simulink model "mdl_4reac_2pump_arduino"  (R2020b)
settings: Solver=FixedStepAuto  StartTime=0.0  StopTime=1000  FixedStep=h  MaxStep=1  RelTol=1e-3  AbsTol=1e-6
undefined symbols (not defined in the file): p_4reac_2pump
settings Model: SILPILModeSetting=veronly  PacingRate=0.100000  ExtModeTrigDuration=2  Creator=nobel  LastModifiedBy=natha
settings OptimizationCC: EnhancedBackFolding=on  PassReuseOutputArgsAs=Individual arguments  ZeroExternalMemoryAtStartup=off  ZeroInternalMemoryAtStartup=off  MaxStackSize=64  OptimizeBlockOrder=speed  DifferentSizesBufferReuse=on  OptimizationCustomize=off  EfficientTunableParamExpr=on
settings DebuggingCC: ParameterTunabilityLossMsg=error
settings HardwareCC: ProdBitPerInt=16  ProdBitPerPointer=16  ProdBitPerSizeT=16  ProdBitPerPtrDiffT=16  ProdLargestAtomicFloat=None  ProdWordSize=8  ProdHWDeviceType=Atmel->AVR  UseEmbeddedCoderFeatures=off  UseSimulinkCoderFeatures=off
settings SFSimCC: MATLABDynamicMemAlloc=off
settings RTWCC: Description=Embedded Coder  SystemTargetFile=ert.tlc  HardwareBoard=Arduino Mega 2560  TemplateMakefile=ert_default_tmf  Toolchain=Arduino AVR
settings CodeAppCC: ForceParamTrailComments=on  IgnoreCustomStorageClasses=off  OperatorAnnotations=on  SimulinkDataObjDesc=on  SFDataObjDesc=on  InsertBlockDesc=on
settings ERTTargetCC: SupportContinuousTime=on  SupportNonInlinedSFcns=on  SupportVariableSizeSignals=on  ExtModeStaticAllocSize=2048

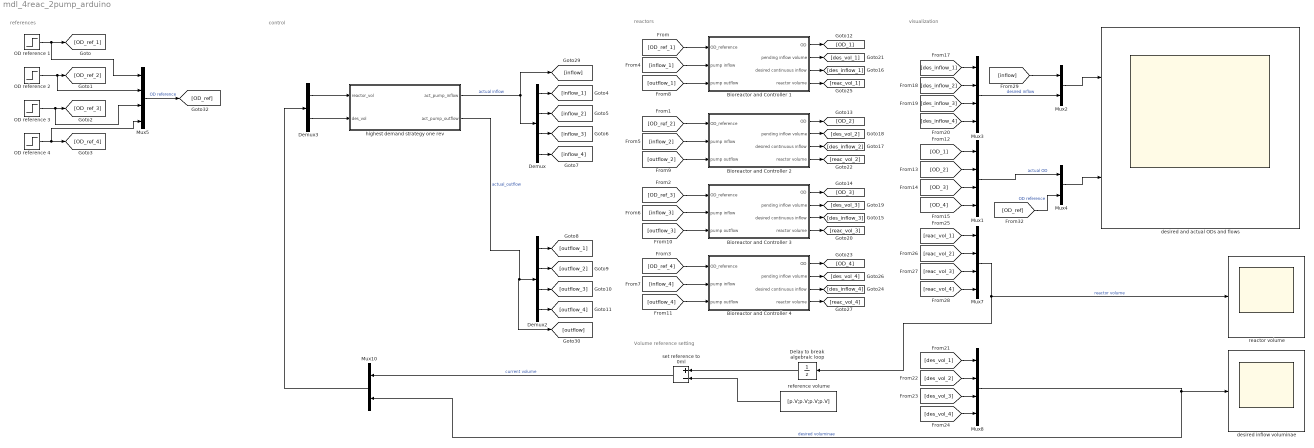
== system mdl_4reac_2pump_arduino ==
  note: control
  note: Volume reference setting
  note: visualization
  note: reactors
  note: references
  Bioreactor and Controller 1 : Subsystem  mask{p=p_4reac_2pump}
      mask prompts: p "Reactor Parameter Struct"
  Bioreactor and Controller 2 : Subsystem  mask{p=p_4reac_2pump}
      mask prompts: p "Reactor Parameter Struct"
  Bioreactor and Controller 3 : Subsystem  mask{p=p_4reac_2pump}
      mask prompts: p "Reactor Parameter Struct"
  Bioreactor and Controller 4 : Subsystem  mask{p=p_4reac_2pump}
      mask prompts: p "Reactor Parameter Struct"
  Delay to break algebraic loop : UnitDelay  InitialCondition=[15; 15; 15; 15]  SampleTime=-1  HasFrameUpgradeWarning=on
  Demux : Demux
  Demux2 : Demux
  Demux3 : Demux  Outputs=2
  Mux{1,3,5,7..8} (5 alike) : Mux
  Mux10 : Mux  Inputs=2
  Mux2 : Mux  Inputs=2
  Mux4 : Mux  Inputs=2
  OD reference 1 : Step  Time=p.r1.step_time  Before=p.r1.init_val  After=p.r1.final_val  SampleTime=0  mask{p=p_4reac_2pump}
      mask prompts: p "Reactor Parameter Struct"
  OD reference 2 : Step  Time=p.r2.step_time  Before=p.r2.init_val  After=p.r2.final_val  SampleTime=0  mask{p=p_4reac_2pump}
      mask prompts: p "Reactor Parameter Struct"
  OD reference 3 : Step  Time=p.r3.step_time  Before=p.r3.init_val  After=p.r3.final_val  SampleTime=0  mask{p=p_4reac_2pump}
      mask prompts: p "Reactor Parameter Struct"
  OD reference 4 : Step  Time=p.r4.step_time  Before=p.r4.init_val  After=p.r4.final_val  SampleTime=0  mask{p=p_4reac_2pump}
      mask prompts: p "Reactor Parameter Struct"
  desired and actual ODs and flows : Scope  NumInputPorts=2
  desired inflow voluminae : Scope
  highest demand strategy one rev : Stateflow chart  TreatAsAtomicUnit=on  mask{p=p_4reac_2pump}
      mask prompts: p "Reactor Parameter Struct"
  reactor volume : Scope
  reference volume : Constant  Value=[p.V;p.V;p.V;p.V]  mask{p=p_4reac_2pump}
      mask prompts: p "Reactor Parameter Struct"
  set reference to 0ml : Sum  Inputs=+-
  wires:
  Bioreactor and Controller 1/2(pending inflow volume) -> [des_vol_1]
  Mux8/1 -> Mux10/2, desired inflow voluminae/1  "desired voluminae"
  Mux1/1 -> Mux4/1  "actual OD"
  Mux2/1 -> desired and actual ODs and flows/1
  Mux3/1 -> Mux2/2  "desired inflow"
  Mux4/1 -> desired and actual ODs and flows/2
  Mux5/1 -> [OD_ref]  "OD reference"
  highest demand strategy one rev/1(act_pump_inflow) -> Demux/1, [inflow]  "actual inflow"
  Mux7/1 -> Delay to break algebraic loop/1, reactor volume/1  "reactor volume"
  reference volume/1 -> set reference to 0ml/2
  OD reference 1/1 -> Mux5/1, [OD_ref_1]
  OD reference 2/1 -> Mux5/2, [OD_ref_2]
  OD reference 3/1 -> Mux5/3, [OD_ref_3]
  OD reference 4/1 -> Mux5/4, [OD_ref_4]
  [OD_ref_1] -> Bioreactor and Controller 1/1(OD_reference)
  [OD_ref_2] -> Bioreactor and Controller 2/1(OD_reference)
  [OD_ref_3] -> Bioreactor and Controller 3/1(OD_reference)
  [OD_ref_4] -> Bioreactor and Controller 4/1(OD_reference)
  Demux/1 -> [inflow_1]
  Demux/2 -> [inflow_2]
  Demux/3 -> [inflow_3]
  Demux/4 -> [inflow_4]
  [inflow_1] -> Bioreactor and Controller 1/2(pump inflow)
  [inflow_2] -> Bioreactor and Controller 2/2(pump inflow)
  [inflow_3] -> Bioreactor and Controller 3/2(pump inflow)
  [inflow_4] -> Bioreactor and Controller 4/2(pump inflow)
  Demux2/4 -> [outflow_4]
  Demux2/3 -> [outflow_3]
  Demux2/2 -> [outflow_2]
  Demux2/1 -> [outflow_1]
  [outflow_1] -> Bioreactor and Controller 1/3(pump outflow)
  [outflow_2] -> Bioreactor and Controller 2/3(pump outflow)
  [outflow_3] -> Bioreactor and Controller 3/3(pump outflow)
  [outflow_4] -> Bioreactor and Controller 4/3(pump outflow)
  Bioreactor and Controller 1/1(OD) -> [OD_1]
  [OD_1] -> Mux1/1
  [OD_2] -> Mux1/2
  [OD_3] -> Mux1/3
  [OD_4] -> Mux1/4
  [des_inflow_1] -> Mux3/1
  [des_inflow_2] -> Mux3/2
  [des_inflow_3] -> Mux3/3
  [des_inflow_4] -> Mux3/4
  [des_vol_4] -> Mux8/4
  [des_vol_3] -> Mux8/3
  [des_vol_2] -> Mux8/2
  [des_vol_1] -> Mux8/1
  Bioreactor and Controller 1/4(reactor volume) -> [reac_vol_1]
  [reac_vol_1] -> Mux7/1
  [reac_vol_2] -> Mux7/2
  [reac_vol_3] -> Mux7/3
  [reac_vol_4] -> Mux7/4
  highest demand strategy one rev/2(act_pump_outflow) -> [outflow], Demux2/1  "actual_outflow"
  [inflow] -> Mux2/1
  [OD_ref] -> Mux4/2  "OD reference"
  set reference to 0ml/1 -> Mux10/1  "current volume"
  Delay to break algebraic loop/1 -> set reference to 0ml/1
  Bioreactor and Controller 1/3(desired continuous inflow) -> [des_inflow_1]
  Bioreactor and Controller 2/3(desired continuous inflow) -> [des_inflow_2]
  Bioreactor and Controller 2/4(reactor volume) -> [reac_vol_2]
  Bioreactor and Controller 2/1(OD) -> [OD_2]
  Bioreactor and Controller 2/2(pending inflow volume) -> [des_vol_2]
  Bioreactor and Controller 3/2(pending inflow volume) -> [des_vol_3]
  Bioreactor and Controller 3/1(OD) -> [OD_3]
  Bioreactor and Controller 3/4(reactor volume) -> [reac_vol_3]
  Bioreactor and Controller 3/3(desired continuous inflow) -> [des_inflow_3]
  Bioreactor and Controller 4/3(desired continuous inflow) -> [des_inflow_4]
  Bioreactor and Controller 4/4(reactor volume) -> [reac_vol_4]
  Bioreactor and Controller 4/1(OD) -> [OD_4]
  Bioreactor and Controller 4/2(pending inflow volume) -> [des_vol_4]
  Demux3/1 -> highest demand strategy one rev/1(reactor_vol)
  Demux3/2 -> highest demand strategy one rev/2(des_vol)
  Mux10/1 -> Demux3/1

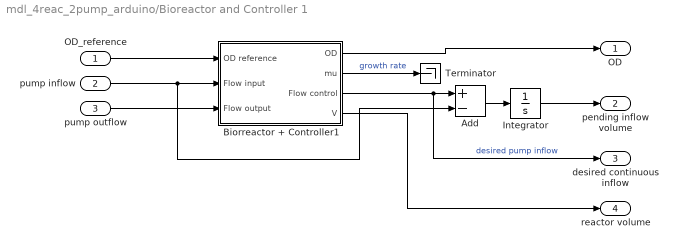
== system mdl_4reac_2pump_arduino/Bioreactor and Controller 1 ==
  OD_reference : Inport
  pump inflow : Inport  Port=2
  pump outflow : Inport  Port=3
  Add : Sum  Inputs=+-
  Biorreactor + Controller1 : Subsystem
  Integrator : Integrator
  Terminator : Terminator
  OD : Outport
  pending inflow volume : Outport  Port=2
  desired continuous inflow : Outport  Port=3
  reactor volume : Outport  Port=4
  wires:
  OD_reference/1 -> Biorreactor + Controller1/1(OD reference)
  Biorreactor + Controller1/2(mu) -> Terminator/1  "growth rate"
  Biorreactor + Controller1/1(OD) -> OD/1
  Biorreactor + Controller1/3(Flow control) -> desired continuous inflow/1, Add/1  "desired pump inflow"
  pump inflow/1 -> Add/2, Biorreactor + Controller1/2(Flow input)
  Biorreactor + Controller1/4(V) -> reactor volume/1
  pump outflow/1 -> Biorreactor + Controller1/3(Flow output)
  Add/1 -> Integrator/1
  Integrator/1 -> pending inflow volume/1

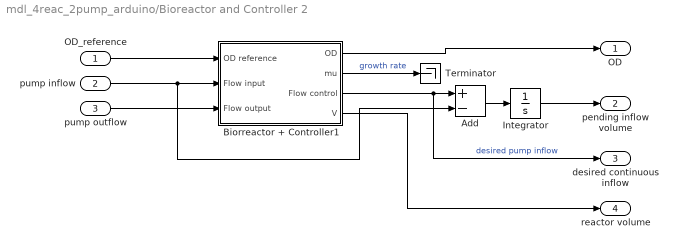
== system mdl_4reac_2pump_arduino/Bioreactor and Controller 2 ==
  OD_reference : Inport
  pump inflow : Inport  Port=2
  pump outflow : Inport  Port=3
  Add : Sum  Inputs=+-
  Biorreactor + Controller1 : Subsystem
  Integrator : Integrator
  Terminator : Terminator
  OD : Outport
  pending inflow volume : Outport  Port=2
  desired continuous inflow : Outport  Port=3
  reactor volume : Outport  Port=4
  wires:
  Integrator/1 -> pending inflow volume/1
  Add/1 -> Integrator/1
  pump outflow/1 -> Biorreactor + Controller1/3(Flow output)
  Biorreactor + Controller1/4(V) -> reactor volume/1
  pump inflow/1 -> Biorreactor + Controller1/2(Flow input), Add/2
  Biorreactor + Controller1/3(Flow control) -> Add/1, desired continuous inflow/1  "desired pump inflow"
  Biorreactor + Controller1/1(OD) -> OD/1
  Biorreactor + Controller1/2(mu) -> Terminator/1  "growth rate"
  OD_reference/1 -> Biorreactor + Controller1/1(OD reference)

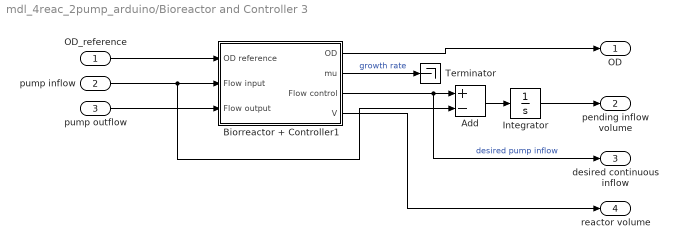
== system mdl_4reac_2pump_arduino/Bioreactor and Controller 3 ==
  OD_reference : Inport
  pump inflow : Inport  Port=2
  pump outflow : Inport  Port=3
  Add : Sum  Inputs=+-
  Biorreactor + Controller1 : Subsystem
  Integrator : Integrator
  Terminator : Terminator
  OD : Outport
  pending inflow volume : Outport  Port=2
  desired continuous inflow : Outport  Port=3
  reactor volume : Outport  Port=4
  wires:
  OD_reference/1 -> Biorreactor + Controller1/1(OD reference)
  Biorreactor + Controller1/2(mu) -> Terminator/1  "growth rate"
  Biorreactor + Controller1/1(OD) -> OD/1
  Biorreactor + Controller1/3(Flow control) -> desired continuous inflow/1, Add/1  "desired pump inflow"
  pump inflow/1 -> Add/2, Biorreactor + Controller1/2(Flow input)
  Biorreactor + Controller1/4(V) -> reactor volume/1
  pump outflow/1 -> Biorreactor + Controller1/3(Flow output)
  Add/1 -> Integrator/1
  Integrator/1 -> pending inflow volume/1

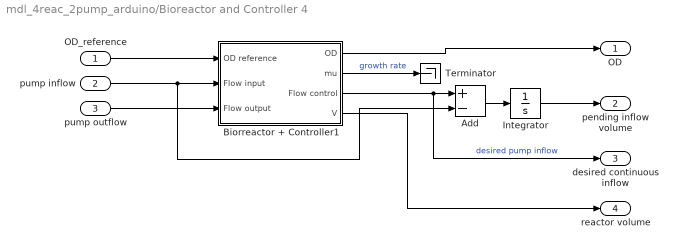
== system mdl_4reac_2pump_arduino/Bioreactor and Controller 4 ==
  OD_reference : Inport
  pump inflow : Inport  Port=2
  pump outflow : Inport  Port=3
  Add : Sum  Inputs=+-
  Biorreactor + Controller1 : Subsystem
  Integrator : Integrator
  Terminator : Terminator
  OD : Outport
  pending inflow volume : Outport  Port=2
  desired continuous inflow : Outport  Port=3
  reactor volume : Outport  Port=4
  wires:
  Integrator/1 -> pending inflow volume/1
  Add/1 -> Integrator/1
  pump outflow/1 -> Biorreactor + Controller1/3(Flow output)
  Biorreactor + Controller1/4(V) -> reactor volume/1
  pump inflow/1 -> Biorreactor + Controller1/2(Flow input), Add/2
  Biorreactor + Controller1/3(Flow control) -> Add/1, desired continuous inflow/1  "desired pump inflow"
  Biorreactor + Controller1/1(OD) -> OD/1
  Biorreactor + Controller1/2(mu) -> Terminator/1  "growth rate"
  OD_reference/1 -> Biorreactor + Controller1/1(OD reference)

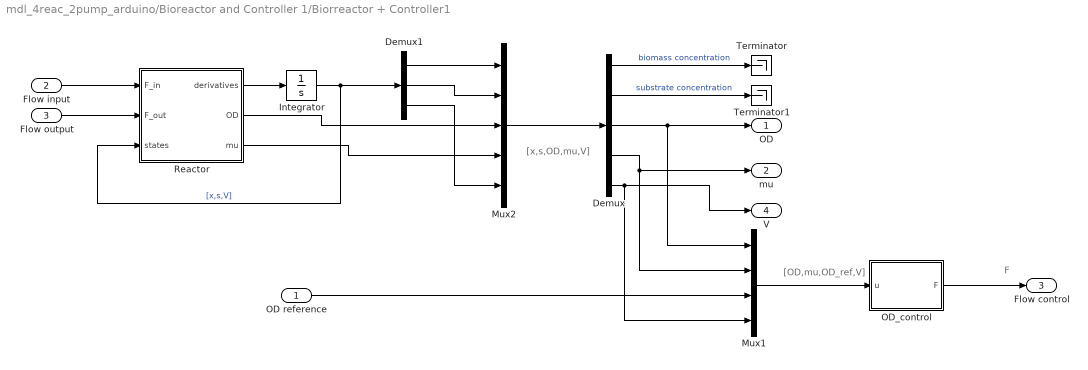
== system mdl_4reac_2pump_arduino/Bioreactor and Controller 1/Biorreactor + Controller1 ==
  note: [OD,mu,OD_ref,V]
  note: F
  note: [x,s,OD,mu,V]
  OD reference : Inport
  Flow input : Inport  Port=2
  Flow output : Inport  Port=3
  Demux : Demux  Outputs=5
  Demux1 : Demux  Outputs=3
  Integrator : Integrator  InitialCondition=[0.1 16 15]
  Mux1 : Mux
  Mux2 : Mux  Inputs=5
  OD_control : MATLAB Function  TreatAsAtomicUnit=on
  Reactor : MATLAB Function  TreatAsAtomicUnit=on
  Terminator : Terminator
  Terminator1 : Terminator
  OD : Outport
  mu : Outport  Port=2
  Flow control : Outport  Port=3
  V : Outport  Port=4
  wires:
  Demux/4 -> Mux1/2, mu/1
  Demux/3 -> Mux1/1, OD/1
  OD reference/1 -> Mux1/3
  Mux2/1 -> Demux/1
  Demux/2 -> Terminator1/1  "substrate concentration"
  Mux1/1 -> OD_control/1(u)
  OD_control/1(F) -> Flow control/1
  Demux/1 -> Terminator/1  "biomass concentration"
  Demux/5 -> Mux1/4, V/1
  Flow output/1 -> Reactor/2(F_out)
  Reactor/1(derivatives) -> Integrator/1
  Integrator/1 -> Demux1/1, Reactor/3(states)  "[x,s,V]"
  Demux1/1 -> Mux2/1
  Demux1/2 -> Mux2/2
  Demux1/3 -> Mux2/5
  Reactor/2(OD) -> Mux2/3
  Reactor/3(mu) -> Mux2/4
  Flow input/1 -> Reactor/1(F_in)

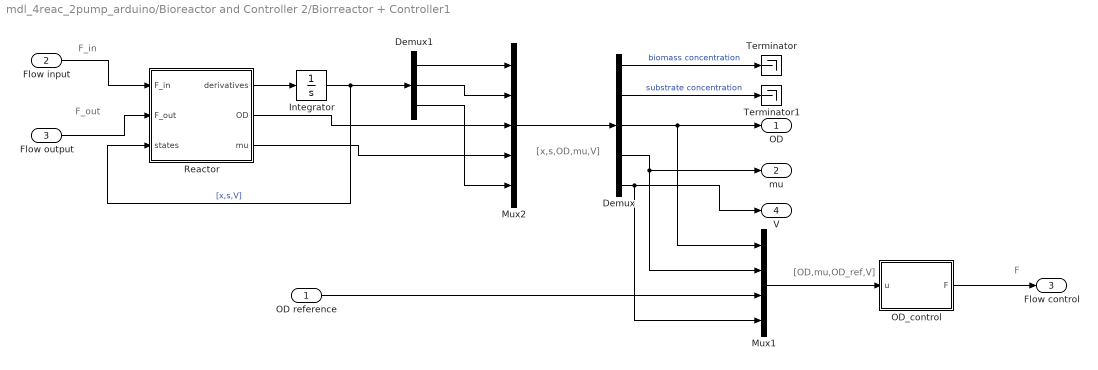
== system mdl_4reac_2pump_arduino/Bioreactor and Controller 2/Biorreactor + Controller1 ==
  note: F_in
  note: [x,s,OD,mu,V]
  note: F
  note: [OD,mu,OD_ref,V]
  note: F_out
  OD reference : Inport
  Flow input : Inport  Port=2
  Flow output : Inport  Port=3
  Demux : Demux  Outputs=5
  Demux1 : Demux  Outputs=3
  Integrator : Integrator  InitialCondition=[0.1 16 15]
  Mux1 : Mux
  Mux2 : Mux  Inputs=5
  OD_control : MATLAB Function  TreatAsAtomicUnit=on
  Reactor : MATLAB Function  TreatAsAtomicUnit=on
  Terminator : Terminator
  Terminator1 : Terminator
  OD : Outport
  mu : Outport  Port=2
  Flow control : Outport  Port=3
  V : Outport  Port=4
  wires:
  Flow input/1 -> Reactor/1(F_in)
  Reactor/3(mu) -> Mux2/4
  Reactor/2(OD) -> Mux2/3
  Demux1/3 -> Mux2/5
  Demux1/2 -> Mux2/2
  Demux1/1 -> Mux2/1
  Integrator/1 -> Reactor/3(states), Demux1/1  "[x,s,V]"
  Reactor/1(derivatives) -> Integrator/1
  Flow output/1 -> Reactor/2(F_out)
  Demux/5 -> V/1, Mux1/4
  Demux/1 -> Terminator/1  "biomass concentration"
  OD_control/1(F) -> Flow control/1
  Mux1/1 -> OD_control/1(u)
  Demux/2 -> Terminator1/1  "substrate concentration"
  Mux2/1 -> Demux/1
  OD reference/1 -> Mux1/3
  Demux/3 -> OD/1, Mux1/1
  Demux/4 -> mu/1, Mux1/2

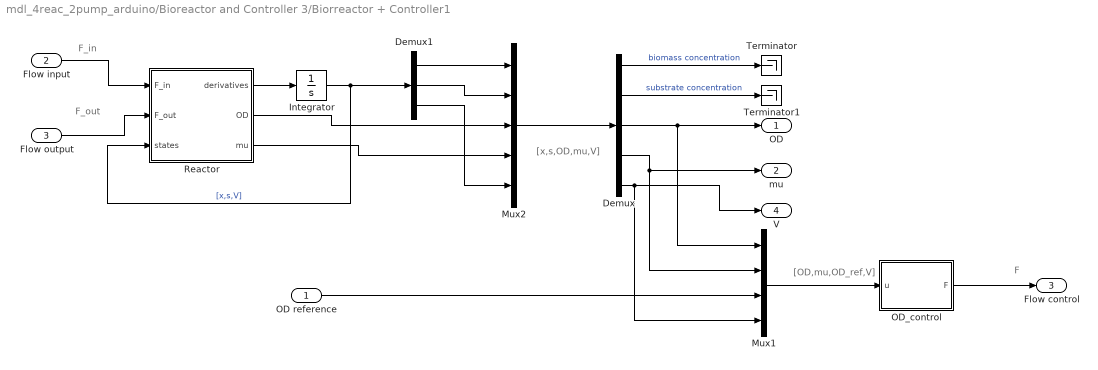
== system mdl_4reac_2pump_arduino/Bioreactor and Controller 3/Biorreactor + Controller1 ==
  note: F_out
  note: [OD,mu,OD_ref,V]
  note: F
  note: [x,s,OD,mu,V]
  note: F_in
  OD reference : Inport
  Flow input : Inport  Port=2
  Flow output : Inport  Port=3
  Demux : Demux  Outputs=5
  Demux1 : Demux  Outputs=3
  Integrator : Integrator  InitialCondition=[0.1 16 15]
  Mux1 : Mux
  Mux2 : Mux  Inputs=5
  OD_control : MATLAB Function  TreatAsAtomicUnit=on
  Reactor : MATLAB Function  TreatAsAtomicUnit=on
  Terminator : Terminator
  Terminator1 : Terminator
  OD : Outport
  mu : Outport  Port=2
  Flow control : Outport  Port=3
  V : Outport  Port=4
  wires:
  Demux/4 -> Mux1/2, mu/1
  Demux/3 -> Mux1/1, OD/1
  OD reference/1 -> Mux1/3
  Mux2/1 -> Demux/1
  Demux/2 -> Terminator1/1  "substrate concentration"
  Mux1/1 -> OD_control/1(u)
  OD_control/1(F) -> Flow control/1
  Demux/1 -> Terminator/1  "biomass concentration"
  Demux/5 -> Mux1/4, V/1
  Flow output/1 -> Reactor/2(F_out)
  Reactor/1(derivatives) -> Integrator/1
  Integrator/1 -> Demux1/1, Reactor/3(states)  "[x,s,V]"
  Demux1/1 -> Mux2/1
  Demux1/2 -> Mux2/2
  Demux1/3 -> Mux2/5
  Reactor/2(OD) -> Mux2/3
  Reactor/3(mu) -> Mux2/4
  Flow input/1 -> Reactor/1(F_in)

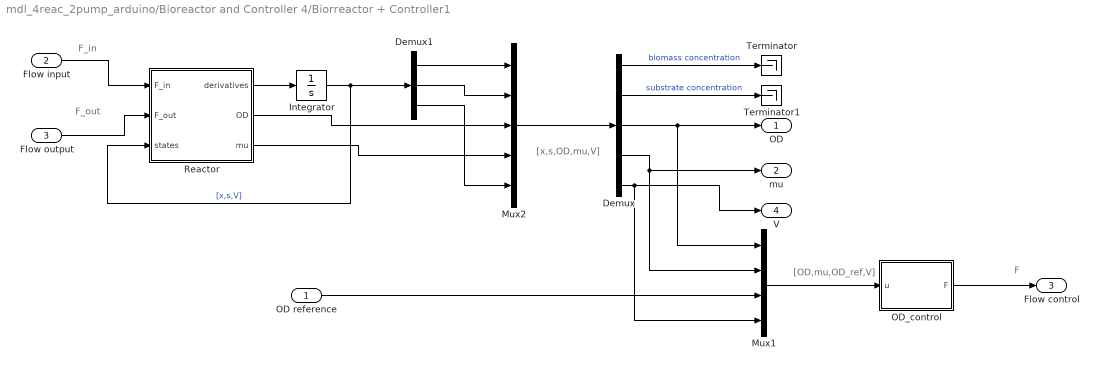
== system mdl_4reac_2pump_arduino/Bioreactor and Controller 4/Biorreactor + Controller1 ==
  note: F_in
  note: [x,s,OD,mu,V]
  note: F
  note: [OD,mu,OD_ref,V]
  note: F_out
  OD reference : Inport
  Flow input : Inport  Port=2
  Flow output : Inport  Port=3
  Demux : Demux  Outputs=5
  Demux1 : Demux  Outputs=3
  Integrator : Integrator  InitialCondition=[0.1 16 15]
  Mux1 : Mux
  Mux2 : Mux  Inputs=5
  OD_control : MATLAB Function  TreatAsAtomicUnit=on
  Reactor : MATLAB Function  TreatAsAtomicUnit=on
  Terminator : Terminator
  Terminator1 : Terminator
  OD : Outport
  mu : Outport  Port=2
  Flow control : Outport  Port=3
  V : Outport  Port=4
  wires:
  Flow input/1 -> Reactor/1(F_in)
  Reactor/3(mu) -> Mux2/4
  Reactor/2(OD) -> Mux2/3
  Demux1/3 -> Mux2/5
  Demux1/2 -> Mux2/2
  Demux1/1 -> Mux2/1
  Integrator/1 -> Reactor/3(states), Demux1/1  "[x,s,V]"
  Reactor/1(derivatives) -> Integrator/1
  Flow output/1 -> Reactor/2(F_out)
  Demux/5 -> V/1, Mux1/4
  Demux/1 -> Terminator/1  "biomass concentration"
  OD_control/1(F) -> Flow control/1
  Mux1/1 -> OD_control/1(u)
  Demux/2 -> Terminator1/1  "substrate concentration"
  Mux2/1 -> Demux/1
  OD reference/1 -> Mux1/3
  Demux/3 -> OD/1, Mux1/1
  Demux/4 -> mu/1, Mux1/2

== stateflow chart mdl_4reac_2pump_arduino/highest demand strategy one rev ==
  state procedures [parallel]
    settings: executionOrder=1
    state normal
    state sampling
      entry: sampling_req=true;
    (default) -> normal
    normal -> sampling : after(15, sec)
    sampling -> normal : sampling_done
  state feeding [parallel]
    settings: executionOrder=2
    state inflow
      state inflow_act
        entry: act_pump_inflow(reac_ind_inflow)=...
        p.max_pump_flow;
      state inflow_inact
        entry: act_pump_inflow=zeros(4,1);
        [vol_pump_in, reac_ind_inflow] = max(des_vol);
        during: [vol_pump_in, reac_ind_inflow] = max(des_vol);
      inflow_act -> inflow_inact : after(p.pump_res/p.max_pump_flow,sec)
      inflow_inact -> inflow_act : [vol_pump_in>=p.pump_res]
    (default) -> inflow_inact
  state wasting_sampling [parallel]
    settings: executionOrder=3
    state outflow_waste
      state outflow_act
        entry: act_pump_outflow(reac_ind_outflow)=...
        p.max_pump_flow;
      state outflow_inact
        entry: act_pump_outflow=zeros(4,1);
        [vol_pump_out, reac_ind_outflow] = max(reactor_vol);
        during: [vol_pump_out, reac_ind_outflow] = ...
        max(reactor_vol);
      wasting_sampling.outflow_waste.outflow_act -> wasting_sampling.outflow_waste.outflow_inact [order 1] : after(vol_pump_out/p.max_pump_flow,sec)
      wasting_sampling.outflow_waste.outflow_act -> wasting_sampling.outflow_waste.outflow_inact [order 2] : [vol_pump_out<=0]
      wasting_sampling.outflow_waste.outflow_inact -> wasting_sampling.outflow_waste.outflow_act [order 2] : [vol_pump_out>=p.pump_res]
    state cleaning_procedure
    state outflow_sampling
      state outflow_act
        entry: vol_pump_out=p.pump_res;
        act_pump_outflow(reac_ind_outflow)=p.max_pump_flow;
      state outflow_inact
        entry: act_pump_outflow=zeros(4,1);
      wasting_sampling.outflow_sampling.outflow_act -> wasting_sampling.outflow_sampling.outflow_inact : after(vol_pump_out/p.max_pump_flow,sec)
      wasting_sampling.outflow_sampling.outflow_inact -> wasting_sampling.outflow_sampling.outflow_act [order 2] : {reac_ind_outflow=reac_ind_outflow+1;}
    (default) -> wasting_sampling.outflow_waste.outflow_inact
    wasting_sampling.outflow_waste.outflow_inact -> cleaning_procedure [order 1] : [in(procedures.sampling)]
    wasting_sampling.outflow_sampling.outflow_inact -> wasting_sampling.outflow_waste.outflow_inact [order 1] : [reac_ind_outflow==4]{send(sampling_done,procedures)}
    cleaning_procedure -> (junction 263) : after(p.clean_time,sec)
    (junction 263) -> wasting_sampling.outflow_sampling.outflow_act : {reac_ind_outflow=1;}
  data: act_pump_inflow output =[0;0;0;0]; reactor_vol input; des_vol input size=4; vol_pump_in local; act_pump_outflow output =[0;0;0;0]; vol_pump_out local; reac_ind_inflow local =1; sampling_req local; p parameter; reac_ind_outflow local =1
  events: sampling_done local FUNCTION_CALL_EVENT

== matlab function mdl_4reac_2pump_arduino/Bioreactor and Controller 1/Biorreactor + Controller1/Reactor ==
  data: F_in input; derivatives output; F_out input; states input; p parameter; OD output; mu output
function [derivatives, OD, mu] = fcn(F_in,F_out,states, p)

x=states(1);
s=states(2);
V=states(3);

D = F_in/V;
mu = p.mu_max*s/(p.K_s+s);

%dx    (Concentration of biomass in the biorreactor)
dx= mu*x - D*x;

%ds    (Concentration of substrate in the biorreactor)
ds= -p.y*mu*x + D*(p.s_f - s);

%dV    (Volume of liquid inside the biorreactor)
dV= F_in - F_out;

OD=x/p.m_p/p.nOD;


derivatives = [dx ds dV];

== matlab function mdl_4reac_2pump_arduino/Bioreactor and Controller 1/Biorreactor + Controller1/OD_control ==
  data: u input; F output
function F = fcn(u)

OD = u(1);
mu = u(2);
OD_ref = u(3);
V = u(4);

F = OD*mu/OD_ref*V;

== matlab function mdl_4reac_2pump_arduino/Bioreactor and Controller 2/Biorreactor + Controller1/OD_control ==
  data: u input; F output
function F = fcn(u)

OD = u(1);
mu = u(2);
OD_ref = u(3);
V = u(4);

F = OD*mu/OD_ref*V;

== matlab function mdl_4reac_2pump_arduino/Bioreactor and Controller 2/Biorreactor + Controller1/Reactor ==
  data: F_in input; derivatives output; F_out input; states input; p parameter; OD output; mu output
function [derivatives, OD, mu] = fcn(F_in,F_out,states, p)

x=states(1);
s=states(2);
V=states(3);

D = F_in/V;
mu = p.mu_max*s/(p.K_s+s);

%dx    (Concentration of biomass in the biorreactor)
dx= mu*x - D*x;

%ds    (Concentration of substrate in the biorreactor)
ds= -p.y*mu*x + D*(p.s_f - s);

%dV    (Volume of liquid inside the biorreactor)
dV= F_in - F_out;

OD=x/p.m_p/p.nOD;


derivatives = [dx ds dV];

== matlab function mdl_4reac_2pump_arduino/Bioreactor and Controller 3/Biorreactor + Controller1/OD_control ==
  data: u input; F output
function F = fcn(u)

OD = u(1);
mu = u(2);
OD_ref = u(3);
V = u(4);

F = OD*mu/OD_ref*V;

== matlab function mdl_4reac_2pump_arduino/Bioreactor and Controller 3/Biorreactor + Controller1/Reactor ==
  data: F_in input; derivatives output; F_out input; states input; p parameter; OD output; mu output
function [derivatives, OD, mu] = fcn(F_in,F_out,states, p)

x=states(1);
s=states(2);
V=states(3);

D = F_in/V;
mu = p.mu_max*s/(p.K_s+s);

%dx    (Concentration of biomass in the biorreactor)
dx= mu*x - D*x;

%ds    (Concentration of substrate in the biorreactor)
ds= -p.y*mu*x + D*(p.s_f - s);

%dV    (Volume of liquid inside the biorreactor)
dV= F_in - F_out;

OD=x/p.m_p/p.nOD;


derivatives = [dx ds dV];

== matlab function mdl_4reac_2pump_arduino/Bioreactor and Controller 4/Biorreactor + Controller1/OD_control ==
  data: u input; F output
function F = fcn(u)

OD = u(1);
mu = u(2);
OD_ref = u(3);
V = u(4);

F = OD*mu/OD_ref*V;

== matlab function mdl_4reac_2pump_arduino/Bioreactor and Controller 4/Biorreactor + Controller1/Reactor ==
  data: F_in input; derivatives output; F_out input; states input; p parameter; OD output; mu output
function [derivatives, OD, mu] = fcn(F_in,F_out,states, p)

x=states(1);
s=states(2);
V=states(3);

D = F_in/V;
mu = p.mu_max*s/(p.K_s+s);

%dx    (Concentration of biomass in the biorreactor)
dx= mu*x - D*x;

%ds    (Concentration of substrate in the biorreactor)
ds= -p.y*mu*x + D*(p.s_f - s);

%dV    (Volume of liquid inside the biorreactor)
dV= F_in - F_out;

OD=x/p.m_p/p.nOD;


derivatives = [dx ds dV];
